simulink model "ControlModelling"  (R2024b)
settings: Solver=ode45  StartTime=0.0  StopTime=50  FixedStep=0.20  RelTol=1e-3
libraries: slpidlib x2
settings Model: PacingRate=0.500000  Creator=pkavi  LastModifiedBy=pkavi

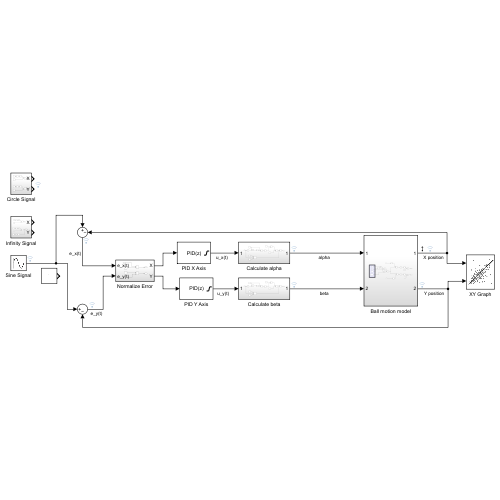
[thumbnail: Simulink's stored preview of the top-level diagram]
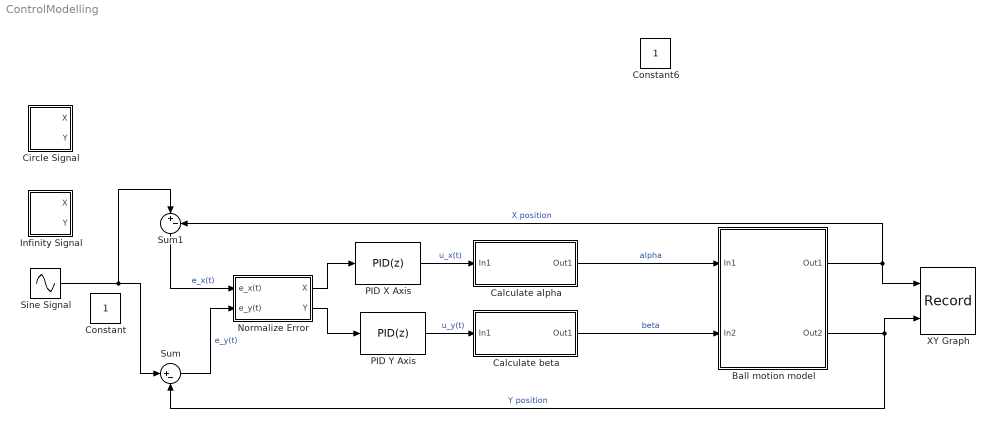
== system ControlModelling ==
  Ball motion model : Subsystem
  Calculate alpha : Subsystem
  Calculate beta : Subsystem
  Circle Signal : Subsystem
  Constant : Constant
  Infinity Signal : Subsystem
  Normalize Error : Subsystem
  PID X Axis : slpidlib/PID Controller  Controller=PID  Form=Parallel  TimeDomain=Discrete-time  UseExternalTs=off  SampleTime=0.020  IntegratorMethod=Forward Euler  FilterMethod=Forward Euler  ControllerParametersSource=internal  P=0.2  I=0.0008  UseKiTs=off  D=0.3  UseExternalDerivativeSource=off  N=1000  UseFilter=off  TunerSelectOption=Transfer Function Based (PID Tuner App)  InitialConditionSource=internal  InitialConditionForIntegrator=0  InitialConditionForFilter=0  DifferentiatorICPrevScaledInput=0  ExternalReset=none  TrackingMode=off  Kt=1  LimitOutput=on  SatLimitsSource=internal  UpperSaturationLimit=0.25  LowerSaturationLimit=-0.25  LinearizeAsGain=off  AntiWindupMode=none  Kb=1  LimitIntegrator=off  UpperIntegratorSaturationLimit=inf  LowerIntegratorSaturationLimit=-inf  POutMin=[]  POutMax=[]  IOutMin=[]  IOutMax=[]  DOutMin=[]  DOutMax=[]  NOutMin=[]  NOutMax=[]  SumOutMin=[]  SumOutMax=[]  SaturationOutMin=[]  SaturationOutMax=[]  PParamMin=[]  PParamMax=[]  IParamMin=[]  IParamMax=[]  DParamMin=[]  DParamMax=[]  NParamMin=[]  NParamMax=[]  KbParamMin=[]  KbParamMax=[]  KtParamMin=[]  KtParamMax=[]  KbOutMin=[]  KbOutMax=[]  KtOutMin=[]  KtOutMax=[]  IntegratorOutMin=[]  IntegratorOutMax=[]  FilterOutMin=[]  FilterOutMax=[]  SumI1OutMin=[]  SumI1OutMax=[]  SumI2OutMin=[]  SumI2OutMax=[]  SumI3OutMin=[]  SumI3OutMax=[]  SumI4OutMin=[]  SumI4OutMax=[]  SumDOutMin=[]  SumDOutMax=[]  DifferentiatorOutMin=[]  DifferentiatorOutMax=[]  FilterDiffOutCoefMin=[]  FilterDiffOutCoefMax=[]  ReciprocalOutMin=[]  ReciprocalOutMax=[]  SumDenOutMin=[]  SumDenOutMax=[]  SumNumOutMin=[]  SumNumOutMax=[]  DivideOutMin=[]  DivideOutMax=[]  UdiffTsProdOutMin=[]  UdiffTsProdOutMax=[]  NTsProdOutMin=[]  NTsProdOutMax=[]  UintegralTsProdOutMin=[]  UintegralTsProdOutMax=[]  UngainTsProdOutMin=[]  UngainTsProdOutMax=[]  ClampingZeroOutDataTypeStr=Inherit: Inherit via back propagation  ClampingZeroOutMin=[]  ClampingZeroOutMax=[]  FilterDenConstantOutDataTypeStr=Inherit: Inherit via back propagation  FilterDenConstantOutMin=[]  FilterDenConstantOutMax=[]  PCopyOutDataTypeStr=Inherit: Inherit via back propagation  PCopyOutMin=[]  PCopyOutMax=[]  NCopyOutDataTypeStr=Inherit: Inherit via back propagation  NCopyOutMin=[]  NCopyOutMax=[]  IntegratorContinuousStateAttributes=''  IntegratorStateMustResolveToSignalObject=off  IntegratorRTWStateStorageClass=Auto  FilterContinuousStateAttributes=''  FilterStateMustResolveToSignalObject=off  FilterRTWStateStorageClass=Auto  ParallelPVariant=InternalParameters  IdealPVariant=Disabled  IVariant=InternalParameters  DVariant=InternalParameters  IntegratorVariant=Discrete  SatVariant=Enabled  AWVariant=Passthrough  PCopyVariant=Disabled  TRVariant=Disabled  FdbkBlocksVariant=Forward  IdealPFdbkVariant=Disabled  SatFdbkVariant=Disabled  DerivativeFilterVariant=Differentiator  NVariant=Passthrough  NCopyVariant=Disabled_SignalSpec  FilterICVariant=InternalICsDifferentiator  IntegratorICVariant=InternalICs  ExternalResetVariant=Disabled  TRSumVariant=Passthrough  SumFdbkVariant=Disabled  SumVariant=Sum_PID  TsampFilterVariant=InternalTs  TsampNgainVariant=Passthrough  TsampIntegralVariant=Disabled_SignalSpec  ExternalSaturationOutDataTypeStr=Inherit: Same as second input  DerivativeSourceVariant=ErrorSignal  PreIntVariant=InternalPreInt
  PID Y Axis : slpidlib/PID Controller  Controller=PID  Form=Parallel  TimeDomain=Discrete-time  UseExternalTs=off  SampleTime=0.020  IntegratorMethod=Forward Euler  FilterMethod=Forward Euler  ControllerParametersSource=internal  P=0.25  I=0  UseKiTs=off  D=0  UseExternalDerivativeSource=off  N=1000  UseFilter=off  TunerSelectOption=Transfer Function Based (PID Tuner App)  InitialConditionSource=internal  InitialConditionForIntegrator=0  InitialConditionForFilter=0  DifferentiatorICPrevScaledInput=0  ExternalReset=none  TrackingMode=off  Kt=1  LimitOutput=on  SatLimitsSource=internal  UpperSaturationLimit=0.25  LowerSaturationLimit=-0.25  LinearizeAsGain=off  AntiWindupMode=none  Kb=1  LimitIntegrator=off  UpperIntegratorSaturationLimit=inf  LowerIntegratorSaturationLimit=-inf  POutMin=[]  POutMax=[]  IOutMin=[]  IOutMax=[]  DOutMin=[]  DOutMax=[]  NOutMin=[]  NOutMax=[]  SumOutMin=[]  SumOutMax=[]  SaturationOutMin=[]  SaturationOutMax=[]  PParamMin=[]  PParamMax=[]  IParamMin=[]  IParamMax=[]  DParamMin=[]  DParamMax=[]  NParamMin=[]  NParamMax=[]  KbParamMin=[]  KbParamMax=[]  KtParamMin=[]  KtParamMax=[]  KbOutMin=[]  KbOutMax=[]  KtOutMin=[]  KtOutMax=[]  IntegratorOutMin=[]  IntegratorOutMax=[]  FilterOutMin=[]  FilterOutMax=[]  SumI1OutMin=[]  SumI1OutMax=[]  SumI2OutMin=[]  SumI2OutMax=[]  SumI3OutMin=[]  SumI3OutMax=[]  SumI4OutMin=[]  SumI4OutMax=[]  SumDOutMin=[]  SumDOutMax=[]  DifferentiatorOutMin=[]  DifferentiatorOutMax=[]  FilterDiffOutCoefMin=[]  FilterDiffOutCoefMax=[]  ReciprocalOutMin=[]  ReciprocalOutMax=[]  SumDenOutMin=[]  SumDenOutMax=[]  SumNumOutMin=[]  SumNumOutMax=[]  DivideOutMin=[]  DivideOutMax=[]  UdiffTsProdOutMin=[]  UdiffTsProdOutMax=[]  NTsProdOutMin=[]  NTsProdOutMax=[]  UintegralTsProdOutMin=[]  UintegralTsProdOutMax=[]  UngainTsProdOutMin=[]  UngainTsProdOutMax=[]  ClampingZeroOutDataTypeStr=Inherit: Inherit via back propagation  ClampingZeroOutMin=[]  ClampingZeroOutMax=[]  FilterDenConstantOutDataTypeStr=Inherit: Inherit via back propagation  FilterDenConstantOutMin=[]  FilterDenConstantOutMax=[]  PCopyOutDataTypeStr=Inherit: Inherit via back propagation  PCopyOutMin=[]  PCopyOutMax=[]  NCopyOutDataTypeStr=Inherit: Inherit via back propagation  NCopyOutMin=[]  NCopyOutMax=[]  IntegratorContinuousStateAttributes=''  IntegratorStateMustResolveToSignalObject=off  IntegratorRTWStateStorageClass=Auto  FilterContinuousStateAttributes=''  FilterStateMustResolveToSignalObject=off  FilterRTWStateStorageClass=Auto  ParallelPVariant=InternalParameters  IdealPVariant=Disabled  IVariant=InternalParameters  DVariant=InternalParameters  IntegratorVariant=Discrete  SatVariant=Enabled  AWVariant=Passthrough  PCopyVariant=Disabled  TRVariant=Disabled  FdbkBlocksVariant=Forward  IdealPFdbkVariant=Disabled  SatFdbkVariant=Disabled  DerivativeFilterVariant=Differentiator  NVariant=Passthrough  NCopyVariant=Disabled_SignalSpec  FilterICVariant=InternalICsDifferentiator  IntegratorICVariant=InternalICs  ExternalResetVariant=Disabled  TRSumVariant=Passthrough  SumFdbkVariant=Disabled  SumVariant=Sum_PID  TsampFilterVariant=InternalTs  TsampNgainVariant=Passthrough  TsampIntegralVariant=Disabled_SignalSpec  ExternalSaturationOutDataTypeStr=Inherit: Same as second input  DerivativeSourceVariant=ErrorSignal  PreIntVariant=InternalPreInt
  Sine Signal : Sin  Amplitude=400  SampleTime=0
  Sum : Sum  Inputs=|+-
  Sum1 : Sum  Inputs=|+-
  XY Graph : Record  FileSettingsInternal="{\"entries\":[{\"content\":{\"excelSettings\":{\"content\":{},\"type\":\"Streamout.ExcelSettings\"}},\"type\":\"Streamout.FileSettingStorage\",\"uuid\":\"\"}],\"packageUris\":[\"http:\\/\\/schema.mathworks.com\\/mf0\\/streamout_blocks\\/R2020a\"],\"version\":\"1.0\"}"  Layout=[1 1]  SignalsInternal="{\"entries\":[{\"content\":{\"signals\":[{\"content\":{\"blockPath\":[],\"dimensions\":[1],\"domain\":\"\",\"lineColor\":\"#a2142f\",\"plots\":[ 1 ],\"port\":1,\"sid\":[\"\"],\"signalID\":1,\"signalName\":\"X position\"},\"type\":\"RecordBlkView.Signal\",\"uuid\":\"\"},{\"content\":{\"blockPath\":[],\"dimensions\":[1],\"domain\":\"\",\"lineColor\":\"#139fff\",\"plots\":[ 1 ],\"port\":2,\"sid\":[\"\"],\"signalID\":2,\"signalName\":\"Y position\"},\"type\":\"RecordBlkView.Signal\",\"uuid\":\"\"}]},\"type\":\"RecordBlkView.InputSignals\",\"uuid\":\"\"}],\"packageUris\":[\"http:\\/\\/schema.mathworks.com\\/mf0\\/streamout_blocks\\/R2020a\"],\"version\":\"1.0\"}"  VisualizationBindings="{\"xyplotplugin\":{\"info\":[{\"series\":[{\"bindingParametersList\":[{\"parameter\":\"X-Axis\",\"signalID\":1,\"signalName\":\"X position\"},{\"parameter\":\"Y-Axis\",\"signalID\":2,\"signalName\":\"Y position\"}],\"seriesID\":0}],\"subplotID\":1}]}}"  CompatibilityTag=XY
  Constant6 : Constant  IOType=siggen
  wires:
  Ball motion model/1(Out1) -> Sum1/2, XY Graph/1  "X position"
  Ball motion model/2(Out2) -> Sum/2, XY Graph/2  "Y position"
  Calculate alpha/1(Out1) -> Ball motion model/1(In1)  "alpha"
  Calculate beta/1(Out1) -> Ball motion model/2(In2)  "beta"
  PID Y Axis/1 -> Calculate beta/1(In1)  "u_y(t)"
  PID X Axis/1 -> Calculate alpha/1(In1)  "u_x(t)"
  Sum1/1 -> Normalize Error/1(e_x(t))  "e_x(t)"
  Sum/1 -> Normalize Error/2(e_y(t))  "e_y(t)"
  Normalize Error/1(X) -> PID X Axis/1
  Normalize Error/2(Y) -> PID Y Axis/1
  Sine Signal/1 -> Sum/1, Sum1/1

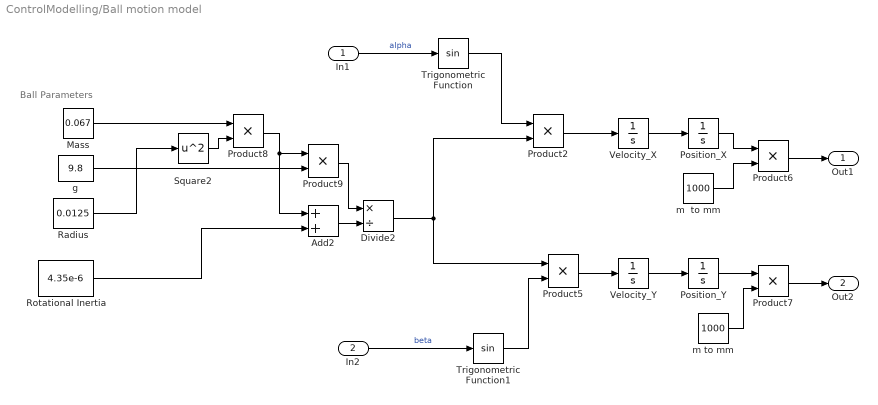
== system ControlModelling/Ball motion model ==
  note: Ball Parameters
  In1 : Inport
  In2 : Inport  Port=2
  Add2 : Sum
  Divide2 : Product  Inputs=*/
  Mass : Constant  Value=0.067
  Position_X : Integrator
  Position_Y : Integrator
  Product{2,5..9} (6 alike) : Product
  Radius : Constant  Value=0.0125
  Rotational Inertia : Constant  Value=4.35e-6
  Square2 : Math  Operator=square
  Trigonometric Function : Trigonometry
  Trigonometric Function1 : Trigonometry
  Velocity_X : Integrator
  Velocity_Y : Integrator
  g : Constant  Value=9.8
  m  to mm : Constant  Value=1000
  m to mm : Constant  Value=1000
  Out1 : Outport
  Out2 : Outport  Port=2
  wires:
  Velocity_Y/1 -> Position_Y/1
  Velocity_X/1 -> Position_X/1
  Product2/1 -> Velocity_X/1
  In1/1 -> Trigonometric Function/1  "alpha"
  In2/1 -> Trigonometric Function1/1  "beta"
  Product5/1 -> Velocity_Y/1
  Trigonometric Function1/1 -> Product5/2
  Trigonometric Function/1 -> Product2/1
  Product6/1 -> Out1/1
  Position_X/1 -> Product6/1
  m  to mm/1 -> Product6/2
  Position_Y/1 -> Product7/1
  m to mm/1 -> Product7/2
  Product7/1 -> Out2/1
  g/1 -> Product9/2
  Mass/1 -> Product8/1
  Radius/1 -> Square2/1
  Rotational Inertia/1 -> Add2/2
  Product9/1 -> Divide2/1
  Add2/1 -> Divide2/2
  Product8/1 -> Add2/1, Product9/1
  Square2/1 -> Product8/2
  Divide2/1 -> Product2/2, Product5/1

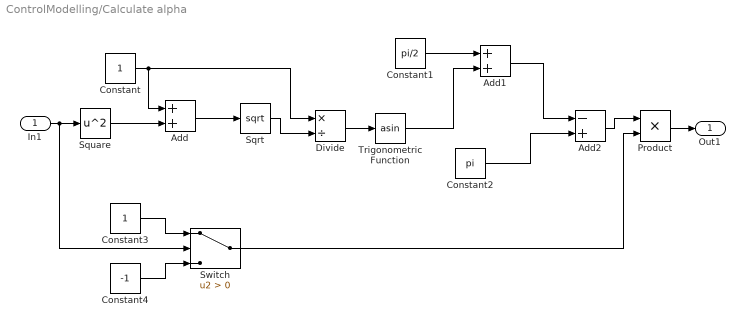
== system ControlModelling/Calculate alpha ==
  In1 : Inport
  Add : Sum
  Add1 : Sum
  Add2 : Sum  Inputs=-+
  Constant : Constant
  Constant1 : Constant  Value=pi/2
  Constant2 : Constant  Value=pi
  Constant3 : Constant
  Constant4 : Constant  Value=-1
  Divide : Product  Inputs=*/
  Product : Product
  Sqrt : Sqrt
  Square : Math  Operator=square
  Switch : Switch  Criteria=u2 > Threshold  SaturateOnIntegerOverflow=off  InputSameDT=off
  Trigonometric Function : Trigonometry  Operator=asin
  Out1 : Outport
  wires:
  In1/1 -> Switch/2, Square/1
  Add/1 -> Sqrt/1
  Sqrt/1 -> Divide/2
  Square/1 -> Add/2
  Constant/1 -> Divide/1, Add/1
  Divide/1 -> Trigonometric Function/1
  Constant1/1 -> Add1/1
  Trigonometric Function/1 -> Add1/2
  Add1/1 -> Add2/1
  Constant2/1 -> Add2/2
  Add2/1 -> Product/1
  Product/1 -> Out1/1
  Constant3/1 -> Switch/1
  Constant4/1 -> Switch/3
  Switch/1 -> Product/2

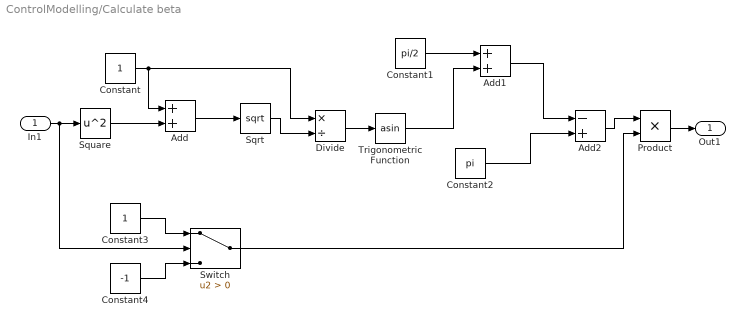
== system ControlModelling/Calculate beta ==
  In1 : Inport
  Add : Sum
  Add1 : Sum
  Add2 : Sum  Inputs=-+
  Constant : Constant
  Constant1 : Constant  Value=pi/2
  Constant2 : Constant  Value=pi
  Constant3 : Constant
  Constant4 : Constant  Value=-1
  Divide : Product  Inputs=*/
  Product : Product
  Sqrt : Sqrt
  Square : Math  Operator=square
  Switch : Switch  Criteria=u2 > Threshold  SaturateOnIntegerOverflow=off  InputSameDT=off
  Trigonometric Function : Trigonometry  Operator=asin
  Out1 : Outport
  wires:
  In1/1 -> Switch/2, Square/1
  Add/1 -> Sqrt/1
  Sqrt/1 -> Divide/2
  Square/1 -> Add/2
  Constant/1 -> Divide/1, Add/1
  Divide/1 -> Trigonometric Function/1
  Constant1/1 -> Add1/1
  Trigonometric Function/1 -> Add1/2
  Add1/1 -> Add2/1
  Constant2/1 -> Add2/2
  Add2/1 -> Product/1
  Product/1 -> Out1/1
  Constant3/1 -> Switch/1
  Constant4/1 -> Switch/3
  Switch/1 -> Product/2

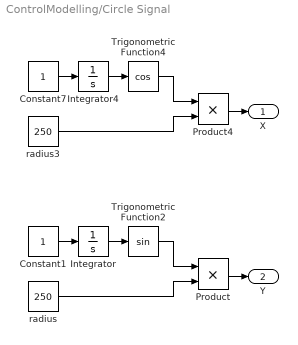
== system ControlModelling/Circle Signal ==
  Constant1 : Constant
  Constant7 : Constant
  Integrator : Integrator
  Integrator4 : Integrator
  Product : Product
  Product4 : Product
  Trigonometric Function2 : Trigonometry
  Trigonometric Function4 : Trigonometry  Operator=cos
  radius : Constant  Value=250
  radius3 : Constant  Value=250
  X : Outport
  Y : Outport  Port=2
  wires:
  Trigonometric Function2/1 -> Product/1
  Trigonometric Function4/1 -> Product4/1
  Integrator4/1 -> Trigonometric Function4/1
  radius3/1 -> Product4/2
  Constant1/1 -> Integrator/1
  Constant7/1 -> Integrator4/1
  Product/1 -> Y/1
  Integrator/1 -> Trigonometric Function2/1
  radius/1 -> Product/2
  Product4/1 -> X/1

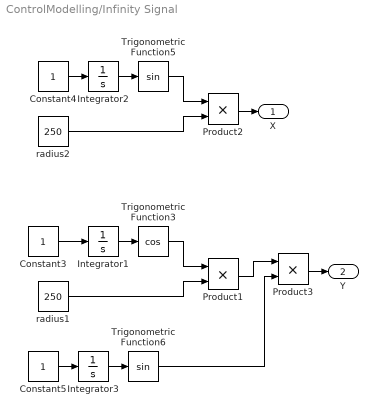
== system ControlModelling/Infinity Signal ==
  Constant3 : Constant
  Constant4 : Constant
  Constant5 : Constant
  Integrator1 : Integrator
  Integrator2 : Integrator
  Integrator3 : Integrator
  Product1 : Product
  Product2 : Product
  Product3 : Product
  Trigonometric Function3 : Trigonometry  Operator=cos
  Trigonometric Function5 : Trigonometry
  Trigonometric Function6 : Trigonometry
  radius1 : Constant  Value=250
  radius2 : Constant  Value=250
  X : Outport
  Y : Outport  Port=2
  wires:
  radius1/1 -> Product1/2
  Integrator1/1 -> Trigonometric Function3/1
  Trigonometric Function5/1 -> Product2/1
  Constant4/1 -> Integrator2/1
  radius2/1 -> Product2/2
  Constant3/1 -> Integrator1/1
  Trigonometric Function6/1 -> Product3/2
  Integrator2/1 -> Trigonometric Function5/1
  Trigonometric Function3/1 -> Product1/1
  Constant5/1 -> Integrator3/1
  Integrator3/1 -> Trigonometric Function6/1
  Product1/1 -> Product3/1
  Product3/1 -> Y/1
  Product2/1 -> X/1

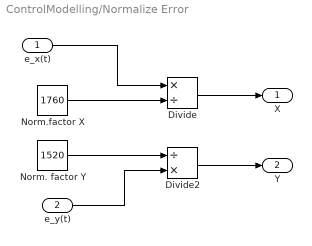
== system ControlModelling/Normalize Error ==
  e_x(t) : Inport
  e_y(t) : Inport  Port=2
  Divide : Product  Inputs=*/
  Divide2 : Product  Inputs=/*
  Norm. factor Y : Constant  Value=1520
  Norm.factor X : Constant  Value=1760
  X : Outport
  Y : Outport  Port=2
  wires:
  Norm.factor X/1 -> Divide/2
  Divide2/1 -> Y/1
  Norm. factor Y/1 -> Divide2/1
  e_y(t)/1 -> Divide2/2
  e_x(t)/1 -> Divide/1
  Divide/1 -> X/1
